simulink model "CT_3"  (Simulink 6.6)
settings: Solver=ode45  StartTime=0.0  StopTime=1e-3  RelTol=1e-3
undefined symbols (not defined in the file): get
libraries: commseqgen2 x1, dspsnks4 x1, commutil2 x1
settings Model: Creator=Мама Люда  LastModifiedBy=Мама Люда  SimulationMode=accelerator

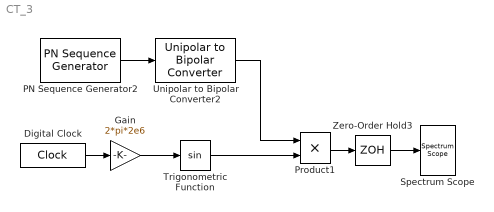
== system CT_3 ==
  Digital Clock : DigitalClock  SampleTime=1e-7
  Gain : Gain  Gain=2*pi*2e6
  PN Sequence Generator2 : commseqgen2/PN Sequence Generator  poly=[1 0 0 0 0 1 0 0 0 1]  ini_sta=[1 1 1 1 1 1 1 0 1]  outBitMaskSource=Dialog parameter  shift=0  Ts=1.955e-6  frameBased=off  sampPerFrame=1  reset=off  bitPackedOutputs=off  outDataType=boolean  numPackedBits=8  bitPackDataSigned=off  bitPackedOutDType=double
  Product1 : Product  RndMeth=Zero
  Spectrum Scope : dspsnks4/Spectrum Scope  DialogController=dspdialog.SpectrumScope  DialogControllerArgs=DataTag0  SystemSampleTime=-1  ScopeProperties=on  Domain=Frequency  HorizSpan=1  UseBuffer=on  BufferSize=1024  Overlap=0  inpFftLenInherit=off  FFTlength=128  numAvg=2  DisplayProperties=off  AxisGrid=on  Memory=off  FrameNumber=on  AxisLegend=off  AxisZoom=off  OpenScopeAtSimStart=on  OpenScopeImmediately=off  FigPos=get(0,'defaultfigureposition')  AxisProperties=off  XUnits=Hertz  XRange=[0...Fs/2]  InheritXIncr=on  XIncr=1.0  XLabel=Samples  XLimit=User-defined  YUnits=dB  XMax=3  XMin=1  YLabel=Magnitude-squared, dB  LineProperties=off  wintypeSpecScope=Bartlett  RsSpecScope=50  betaSpecScope=5  winsampSpecScope=Periodic
      settings: YMin=-31.560815522706  YMax=10.5419195173934
  Trigonometric Function : Trigonometry
  Unipolar to Bipolar Converter2 : commutil2/Unipolar to Bipolar Converter  SystemSampleTime=-1  M=2  polarity=Positive  dataType=double
  Zero-Order Hold3 : ZeroOrderHold  SampleTime=1e-7
  wires:
  Unipolar to Bipolar Converter2/1 -> Product1/1
  PN Sequence Generator2/1 -> Unipolar to Bipolar Converter2/1
  Digital Clock/1 -> Gain/1
  Gain/1 -> Trigonometric Function/1
  Trigonometric Function/1 -> Product1/2
  Zero-Order Hold3/1 -> Spectrum Scope/1
  Product1/1 -> Zero-Order Hold3/1
